simulink model "TPS_Modelslx"  (R2024b)
settings: Solver=VariableStepDiscrete  StartTime=0.0  StopTime=10.0  RelTol=1e-3
settings Model: Creator=Ahmad  LastModifiedBy=Ahmad

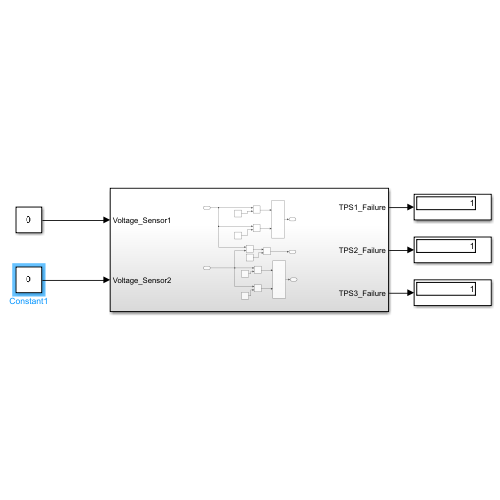
[thumbnail: Simulink's stored preview of the top-level diagram]
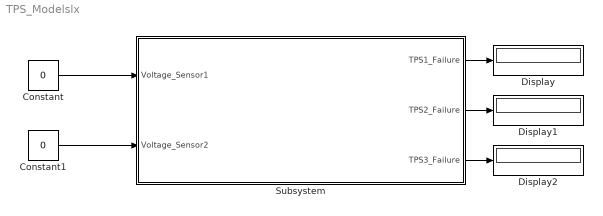
== system TPS_Modelslx ==
  Constant : Constant  Value=0  OutDataTypeStr=single
  Constant1 : Constant  Value=0  OutDataTypeStr=single
  Display : Display
  Display1 : Display
  Display2 : Display
  Subsystem : Subsystem
  wires:
  Constant/1 -> Subsystem/1(Voltage_Sensor1)
  Constant1/1 -> Subsystem/2(Voltage_Sensor2)
  Subsystem/1(TPS1_Failure) -> Display/1
  Subsystem/2(TPS2_Failure) -> Display1/1
  Subsystem/3(TPS3_Failure) -> Display2/1

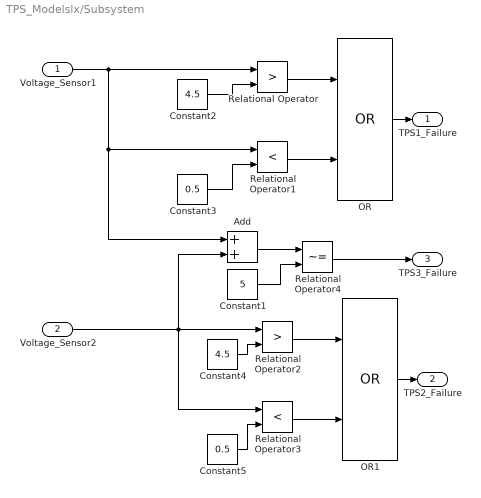
== system TPS_Modelslx/Subsystem ==
  Voltage_Sensor1 : Inport
  Voltage_Sensor2 : Inport  Port=2
  Add : Sum
  Constant1 : Constant  Value=5
  Constant2 : Constant  Value=4.5
  Constant3 : Constant  Value=0.5
  Constant4 : Constant  Value=4.5
  Constant5 : Constant  Value=0.5
  OR : Logic  Operator=OR  AllPortsSameDT=off  OutDataTypeStr=boolean
  OR1 : Logic  Operator=OR  AllPortsSameDT=off  OutDataTypeStr=boolean
  Relational Operator : RelationalOperator  Operator=>  OutDataTypeStr=boolean  RndMeth=Simplest  InputSameDT=off
  Relational Operator1 : RelationalOperator  Operator=<  OutDataTypeStr=boolean  RndMeth=Simplest  InputSameDT=off
  Relational Operator2 : RelationalOperator  Operator=>  OutDataTypeStr=boolean  RndMeth=Simplest  InputSameDT=off
  Relational Operator3 : RelationalOperator  Operator=<  OutDataTypeStr=boolean  RndMeth=Simplest  InputSameDT=off
  Relational Operator4 : RelationalOperator  Operator=~=  OutDataTypeStr=boolean  RndMeth=Simplest  InputSameDT=off
  TPS1_Failure : Outport  OutDataTypeStr=boolean
  TPS2_Failure : Outport  Port=2  OutDataTypeStr=boolean
  TPS3_Failure : Outport  Port=3  OutDataTypeStr=boolean
  wires:
  Constant4/1 -> Relational Operator2/2
  Relational Operator/1 -> OR/1
  Constant2/1 -> Relational Operator/2
  Constant5/1 -> Relational Operator3/2
  Relational Operator3/1 -> OR1/2
  Constant3/1 -> Relational Operator1/2
  Relational Operator2/1 -> OR1/1
  Voltage_Sensor1/1 -> Relational Operator1/1, Add/1, Relational Operator/1
  Voltage_Sensor2/1 -> Relational Operator3/1, Relational Operator2/1, Add/2
  Relational Operator1/1 -> OR/2
  OR1/1 -> TPS2_Failure/1
  OR/1 -> TPS1_Failure/1
  Add/1 -> Relational Operator4/1
  Constant1/1 -> Relational Operator4/2
  Relational Operator4/1 -> TPS3_Failure/1
